simulink model "seldom_sim"  (R2024a)
settings: Solver=FixedStepAuto  StartTime=0.0  StopTime=30  FixedStep=framePeriod_s  RelTol=1e-9
values from neighbouring files (symbols this model uses):
  framePeriod_s = 1/frameRate_hz    (= 0.02)    [setup.m]
undefined symbols (not defined in the file or in its folder): accel_mps2, Aircraft, alt_wgs84_m, ch, current_ma, datetime, datevec, die_temp_c, Earth, Env, ext_gnss1, failsafe, fmu_imu, fmu_mag, frame_time_us, gps_tow_ms, gyro_radps, healthy, horz_acc_m, imu_healthy, inceptor, InitCond, installed, lat_rad, lon_rad, lost_frame, mag_ut, ned_vel_mps, new_data, num_sats, power_module, sys_time_us, Telem, vert_acc_m, voltage_v, week, WGS84
libraries: simulink x8, aerolibconvert2 x5, aerolibasang x3, aerolibtransform2 x2, aerolibgravity2 x2, aerolibatmos2 x1, sharedtransform x1, uavutilslib x1, vrlib x1, simulink_extras x1, spsLeadLagFilterLib x1, shared6dof x1
(part 2 of 2)

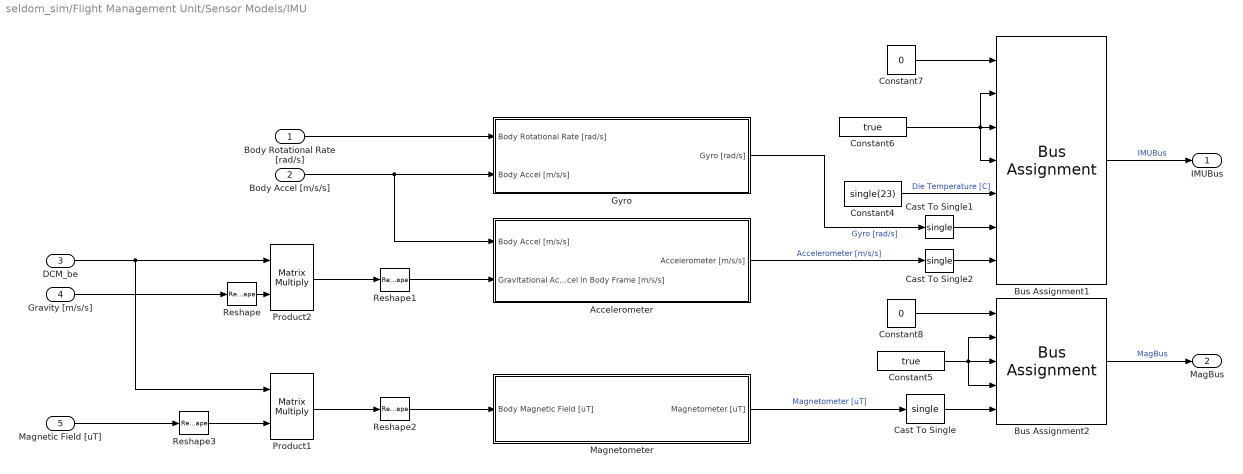
== system seldom_sim/Flight Management Unit/Sensor Models/IMU ==
  Body Rotational Rate [rad/s] : Inport
  Body Accel [m/s/s] : Inport  Port=2
  DCM_be : Inport  Port=3
  Gravity [m/s/s] : Inport  Port=4
  Magnetic Field [uT] : Inport  Port=5
  Accelerometer : Subsystem
  Bus Assignment1 : BusAssignment  AssignedSignals=installed,imu_healthy,new_data,die_temp_c,gyro_radps,accel_mps2
  Bus Assignment2 : BusAssignment  AssignedSignals=installed,healthy,new_data,mag_ut
  Cast To Single : DataTypeConversion  OutDataTypeStr=single  SaturateOnIntegerOverflow=off  RndMeth=Floor
  Cast To Single1 : DataTypeConversion  OutDataTypeStr=single  SaturateOnIntegerOverflow=off  RndMeth=Floor
  Cast To Single2 : DataTypeConversion  OutDataTypeStr=single  SaturateOnIntegerOverflow=off  RndMeth=Floor
  Constant4 : Constant  Value=single(23)
  Constant5 : Constant  Value=true
  Constant6 : Constant  Value=true
  Constant7 : Constant  Value=0  OutDataTypeStr=Bus: ImuData
  Constant8 : Constant  Value=0  OutDataTypeStr=Bus: MagData
  Gyro : Subsystem
  Magnetometer : Subsystem
  Product1 : Product  Multiplication=Matrix(*)
  Product2 : Product  Multiplication=Matrix(*)
  Reshape : Reshape  OutputDimensionality=Column vector (2-D)
  Reshape1 : Reshape
  Reshape2 : Reshape
  Reshape3 : Reshape  OutputDimensionality=Column vector (2-D)
  IMUBus : Outport
  MagBus : Outport  Port=2
  wires:
  Body Accel [m/s/s]/1 -> Accelerometer/1(Body Accel [m/s/s]), Gyro/2(Body Accel [m/s/s])
  DCM_be/1 -> Product1/1, Product2/1
  Gravity [m/s/s]/1 -> Reshape/1
  Product2/1 -> Reshape1/1
  Reshape1/1 -> Accelerometer/2(Gravitational Accel in Body Frame [m/s/s])
  Body Rotational Rate [rad/s]/1 -> Gyro/1(Body Rotational Rate [rad/s])
  Reshape2/1 -> Magnetometer/1(Body Magnetic Field [uT])
  Product1/1 -> Reshape2/1
  Reshape3/1 -> Product1/2
  Magnetic Field [uT]/1 -> Reshape3/1
  Magnetometer/1(Magnetometer [uT]) -> Cast To Single/1  "Magnetometer [uT]"
  Accelerometer/1(Accelerometer [m/s/s]) -> Cast To Single2/1  "Accelerometer [m/s/s]"
  Gyro/1(Gyro [rad/s]) -> Cast To Single1/1  "Gyro [rad/s]"
  Reshape/1 -> Product2/2
  Constant4/1 -> Bus Assignment1/5  "Die Temperature [C]"
  Constant7/1 -> Bus Assignment1/1
  Constant8/1 -> Bus Assignment2/1
  Bus Assignment2/1 -> MagBus/1  "MagBus"
  Bus Assignment1/1 -> IMUBus/1  "IMUBus"
  Constant5/1 -> Bus Assignment2/4, Bus Assignment2/2, Bus Assignment2/3
  Constant6/1 -> Bus Assignment1/4, Bus Assignment1/2, Bus Assignment1/3
  Cast To Single/1 -> Bus Assignment2/5
  Cast To Single1/1 -> Bus Assignment1/6
  Cast To Single2/1 -> Bus Assignment1/7

== system seldom_sim/Flight Management Unit/Sensor Models/MakeInceptorBus ==
  Inceptor : Inport
  Bus Assignment1 : BusAssignment  AssignedSignals=new_data,lost_frame,failsafe,ch
  Bus Selector2 : BusSelector  OutputSignals=New Data,Lost Frame,Failsafe,Channel Data
  Constant4 : Constant  Value=0  OutDataTypeStr=Bus: InceptorData
  InceptorBus : Outport
  wires:
  Bus Selector2/2 -> Bus Assignment1/3  "<Lost Frame>"
  Bus Selector2/1 -> Bus Assignment1/2  "<New Data>"
  Inceptor/1 -> Bus Selector2/1
  Bus Selector2/4 -> Bus Assignment1/5  "<Channel Data>"
  Bus Assignment1/1 -> InceptorBus/1  "InceptorBus"
  Bus Selector2/3 -> Bus Assignment1/4  "<Failsafe>"
  Constant4/1 -> Bus Assignment1/1

== system seldom_sim/Flight Management Unit/Sensor Models/MakePowerModuleBus ==
  Battery : Inport
  Bus Assignment1 : BusAssignment  AssignedSignals=voltage_v,current_ma
  Bus Selector2 : BusSelector  OutputSignals=Voltage [V],Current [V]
  Constant4 : Constant  Value=0  OutDataTypeStr=Bus: PowerModuleData
  PowerModuleBus : Outport
  wires:
  Constant4/1 -> Bus Assignment1/1
  Bus Assignment1/1 -> PowerModuleBus/1  "PowerModuleBus"
  Battery/1 -> Bus Selector2/1
  Bus Selector2/1 -> Bus Assignment1/2  "<Voltage [V]>"
  Bus Selector2/2 -> Bus Assignment1/3  "<Current [V]>"

== system seldom_sim/Flight Management Unit/Subsystem/Triggered Subsystem ==
  Wp : Inport
  Trigger : TriggerPort  VariantControl=(inherit)
  Constant : Constant  OutDataTypeStr=int16
  Sum : Sum  Inputs=|++  AccumDataTypeStr=uint16
  Wp++ : Outport
  wires:
  Wp/1 -> Sum/1
  Constant/1 -> Sum/2
  Sum/1 -> Wp++/1

== system seldom_sim/Vehicle/Forces and Moments/Aerodynamic ==
  note: In the future, the effect of blade flapping will be included. More experimental test need to be done to evaluate the v_forward to deflection angle constant in a wind tunnel.
  note: To calculate drag force, a look up table was created by recording the projected area at different incident angles. Assume the drone to resemble a cylinder (area changes as angle of attack changes, constant with sideslip changes)
  Dynamic Pressure : Inport
  body_vel : Inport  Port=2
  Calculate wind angle : Subsystem
  Cd : Constant  Value=Aircraft.Aero.Cd
  Drag contribution on moment : Constant  Value=[0 0 0]
  Drag in body frame : Product  Multiplication=Matrix(*)
  Gain : Gain  Gain=-1
  Mux1 : Mux  Inputs=2
  Normalize Vector : vrlib/Utilities/Normalize Vector  maxzero=0
  Product : Product  Inputs=3
  Radians to Degrees : simulink_extras/Transformations/Radians to Degrees
  Reshape : Reshape  OutputDimensionality=Row vector (2-D)
  alfa to frontal area look up table : Lookup_n-D  NumberOfTableDimensions=1  BreakpointsSpecification=Even spacing  BreakpointsForDimension1=[-90:10:90]  BreakpointsForDimension1FirstPoint=-180  BreakpointsForDimension1Spacing=10  Table=Aircraft.Geo.front_area_m2  InternalRulePriority=Speed  RndMeth=Simplest
  Fxyz Mxzy : Outport
  wires:
  Dynamic Pressure/1 -> Product/2
  Product/1 -> Drag in body frame/2
  Reshape/1 -> Fxyz Mxzy/1
  Mux1/1 -> Reshape/1
  Radians to Degrees/1 -> alfa to frontal area look up table/1
  alfa to frontal area look up table/1 -> Product/1  "Frontal area"
  Cd/1 -> Product/3
  Drag in body frame/1 -> Mux1/1
  Drag contribution on moment/1 -> Mux1/2
  Gain/1 -> Normalize Vector/1
  Normalize Vector/1 -> Drag in body frame/1
  body_vel/1 -> Gain/1, Calculate wind angle/1(body_vel_mps)
  Calculate wind angle/1(Incident_angle_rad) -> Radians to Degrees/1

== system seldom_sim/Vehicle/Forces and Moments/Gravitational ==
  Gravity [m/s/s] : Inport
  DCM_be : Inport  Port=2
  Gravity Moment : Constant  Value=[0 0 0]
  Mux : Mux  Inputs=2
  Product : Product
  Product1 : Product  Multiplication=Matrix(*)
  Reshape : Reshape  OutputDimensionality=Column vector (2-D)
  Reshape1 : Reshape
  UAV Mass : Constant  Value=Aircraft.Mass.mass_kg
  Fxyz Mxyz : Outport
  wires:
  UAV Mass/1 -> Product/2
  Product/1 -> Product1/2  "Gravity Force NED [N]"
  DCM_be/1 -> Product1/1
  Gravity Moment/1 -> Mux/2
  Mux/1 -> Fxyz Mxyz/1
  Reshape/1 -> Product/1
  Gravity [m/s/s]/1 -> Reshape/1
  Reshape1/1 -> Mux/1
  Product1/1 -> Reshape1/1  "Gravity Force Body [N]"

== system seldom_sim/Vehicle/Forces and Moments/Propulsive ==
  note: Should get replaced with full and proper motor lookup tables unless it is really very linear.
  note: Missing modeling of torque directly generated from the motor plus propeller spinning. Need to add that in.
  note: First order response model of motor thrust to command change.
  Motor Cmd : Inport
  Constant1 : Constant  Value=Aircraft.Motor.align
  Constant7 : Constant  Value=Aircraft.Motor.pos_m
  Demux1 : Demux  Outputs=3
  Demux2 : Demux  Outputs=3
  Gain : Gain  Gain=Aircraft.Motor.fmaxa_N
  Lead-Lag Filter : spsLeadLagFilterLib/Lead-Lag Filter  T1=0  T2=Aircraft.Motor.Tau  Vdc_Init=0  Ts=0
      settings: LibrarySourceBlock=|
      | sps_lib/Control/Filters/Lead-Lag
      | Filter
  Motor_Force_and_Moment_Body : MATLAB Function  TreatAsAtomicUnit=on
  Mux1 : Mux  Inputs=6
  PWM_norm : Subsystem
  Reshape2 : Reshape  OutputDimensionality=Row vector (2-D)
  Reshape3 : Reshape  OutputDimensionality=Row vector (2-D)
  Fxyz Mxyz : Outport
  wires:
  Reshape2/1 -> Motor_Force_and_Moment_Body/3(motor_thrust)
  Motor Cmd/1 -> PWM_norm/1(raw_sbus_in)
  Motor_Force_and_Moment_Body/2(Moment_motor) -> Demux1/1
  Demux1/1 -> Mux1/4  "Mx"
  Demux1/2 -> Mux1/5  "My"
  Constant7/1 -> Motor_Force_and_Moment_Body/1(motor_pos)
  Reshape3/1 -> Fxyz Mxyz/1
  Demux1/3 -> Mux1/6  "Mz"
  Mux1/1 -> Reshape3/1
  Constant1/1 -> Motor_Force_and_Moment_Body/2(motor_align)
  Demux2/2 -> Mux1/2  "Fy"
  Demux2/1 -> Mux1/1  "Fx"
  Demux2/3 -> Mux1/3  "Fz"
  Motor_Force_and_Moment_Body/1(Force_motor) -> Demux2/1
  Lead-Lag Filter/1 -> Gain/1  "PWM_ND_lag"
  Gain/1 -> Reshape2/1
  PWM_norm/1(normalized_out) -> Lead-Lag Filter/1  "PWM_ND"

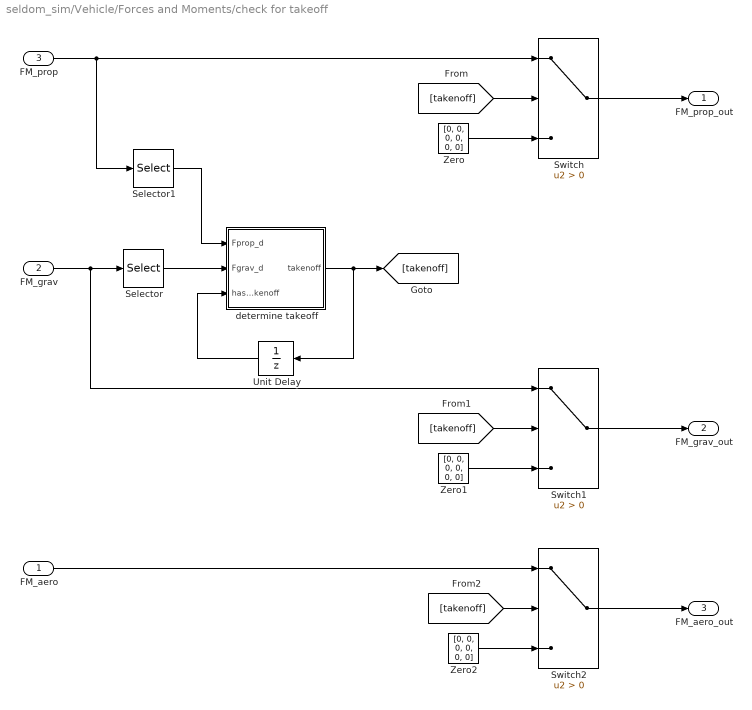
== system seldom_sim/Vehicle/Forces and Moments/check for takeoff ==
  FM_aero : Inport
  FM_grav : Inport  Port=2
  FM_prop : Inport  Port=3
  Selector : Selector  NumberOfDimensions=2  InputPortWidth=3  IndexOptions=Index vector (dialog),Index vector (dialog)  Indices=1,3  OutputSizes=1,1
  Selector1 : Selector  NumberOfDimensions=2  InputPortWidth=3  IndexOptions=Index vector (dialog),Index vector (dialog)  Indices=1,3  OutputSizes=1,1
  Switch : Switch  Criteria=u2 > Threshold  SaturateOnIntegerOverflow=off  InputSameDT=off
  Switch1 : Switch  Criteria=u2 > Threshold  SaturateOnIntegerOverflow=off  InputSameDT=off
  Switch2 : Switch  Criteria=u2 > Threshold  SaturateOnIntegerOverflow=off  InputSameDT=off
  Unit Delay : UnitDelay  InitialCondition=false  SampleTime=-1  HasFrameUpgradeWarning=on
  Zero : Constant  Value=[0, 0, 0, 0, 0, 0]  VectorParams1D=off  OutDataTypeStr=Inherit: Inherit via back propagation
  Zero1 : Constant  Value=[0, 0, 0, 0, 0, 0]  VectorParams1D=off  OutDataTypeStr=Inherit: Inherit via back propagation
  Zero2 : Constant  Value=[0, 0, 0, 0, 0, 0]  VectorParams1D=off  OutDataTypeStr=Inherit: Inherit via back propagation
  determine takeoff : Subsystem
  FM_prop_out : Outport
  FM_grav_out : Outport  Port=2
  FM_aero_out : Outport  Port=3
  wires:
  Switch2/1 -> FM_aero_out/1
  [takenoff] -> Switch1/2
  FM_prop/1 -> Selector1/1, Switch/1
  FM_aero/1 -> Switch2/1
  Switch1/1 -> FM_grav_out/1
  Selector1/1 -> determine takeoff/1(Fprop_d)
  FM_grav/1 -> Selector/1, Switch1/1
  Unit Delay/1 -> determine takeoff/3(has_takenoff)
  determine takeoff/1(takenoff) -> [takenoff], Unit Delay/1
  Zero1/1 -> Switch1/3
  Zero2/1 -> Switch2/3
  Zero/1 -> Switch/3
  Selector/1 -> determine takeoff/2(Fgrav_d)
  [takenoff] -> Switch/2
  [takenoff] -> Switch2/2
  Switch/1 -> FM_prop_out/1

== system seldom_sim/Vehicle/Vehicle Model/Norm ==
  2D Vector : Inport
  Product : Product
  Sqrt : Sqrt
  Sum of Elements : Sum  Inputs=+
  Norm : Outport
  wires:
  2D Vector/1 -> Product/2, Product/1
  Product/1 -> Sum of Elements/1
  Sum of Elements/1 -> Sqrt/1
  Sqrt/1 -> Norm/1

== system seldom_sim/Vehicle/Vehicle Model/determine airespeed ==
  Vb : Inport
  Compare To Constant : simulink/Logic and Bit Operations/Compare To Constant  relop=>  const=0  OutDataTypeStr=boolean
  MatrixMultiply : Product  Multiplication=Matrix(*)
  Reshape : Reshape  OutputDimensionality=Column vector (2-D)
  Reshape1 : Reshape  OutputDimensionality=Row vector (2-D)
  Subsystem : Subsystem
  AoA rate : Outport
  Alpha : Outport  Port=2
  Beta : Outport  Port=3
  beta rate : Outport  Port=4
  airspeed : Outport  Port=5
  wires:
  Vb/1 -> Subsystem/1(Vb), Reshape/1, Reshape1/1
  Reshape1/1 -> MatrixMultiply/1
  Reshape/1 -> MatrixMultiply/2
  MatrixMultiply/1 -> Compare To Constant/1
  Subsystem/1(AoA rate) -> AoA rate/1
  Subsystem/2(Alpha) -> Alpha/1
  Subsystem/3(Beta) -> Beta/1
  Subsystem/4(beta rate) -> beta rate/1
  Subsystem/5(V) -> airspeed/1
  Compare To Constant/1 -> Subsystem/Enable

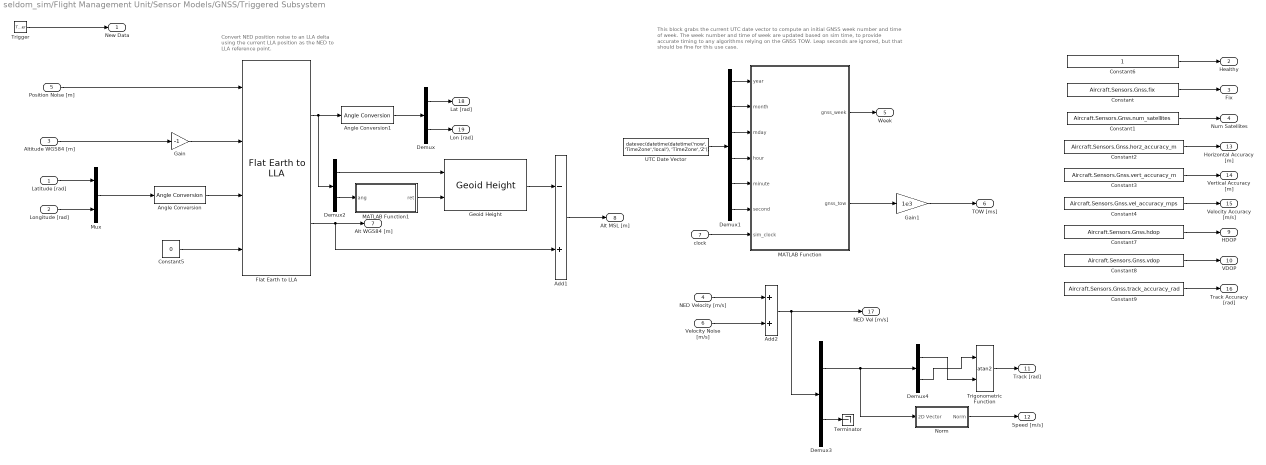
== system seldom_sim/Flight Management Unit/Sensor Models/GNSS/Triggered Subsystem ==
  note: This block grabs the current UTC date vector to compute an initial GNSS week number
      | and time of week. The week number and time of week are updated based on sim time, to provide accurate timing to any algorithms relying on the GNSS TOW. Leap seconds are ignored, but that should be fine for this use case.
  note: Convert NED position noise to an LLA delta
      | using the current LLA position as the NED to
      | LLA reference point.
  Latitude [rad] : Inport
  "Longitude [rad] " : Inport  Port=2
  Altitude WGS84 [m] : Inport  Port=3
  NED Velocity [m/s] : Inport  Port=4  PortDimensions=3
  Position Noise [m] : Inport  Port=5  PortDimensions=3
  Velocity Noise [m/s] : Inport  Port=6  PortDimensions=3
  clock : Inport  Port=7
  Trigger : TriggerPort  VariantControl=Variant  ShowOutputPort=on  OutputDataType=int8
  Add1 : Sum  Inputs=-+
  Add2 : Sum
  Angle Conversion : aerolibconvert2/Angle Conversion  IU=rad  OU=deg
  Angle Conversion1 : aerolibconvert2/Angle Conversion  IU=deg  OU=rad
  Constant : Constant  Value=Aircraft.Sensors.Gnss.fix
  Constant1 : Constant  Value=Aircraft.Sensors.Gnss.num_satellites
  Constant2 : Constant  Value=Aircraft.Sensors.Gnss.horz_accuracy_m
  Constant3 : Constant  Value=Aircraft.Sensors.Gnss.vert_accuracy_m
  Constant4 : Constant  Value=Aircraft.Sensors.Gnss.vel_accuracy_mps
  Constant5 : Constant  Value=0
  Constant6 : Constant
  Constant7 : Constant  Value=Aircraft.Sensors.Gnss.hdop
  Constant8 : Constant  Value=Aircraft.Sensors.Gnss.vdop
  Constant9 : Constant  Value=Aircraft.Sensors.Gnss.track_accuracy_rad
  Demux : Demux  Outputs=2
  Demux1 : Demux  Outputs=6
  Demux2 : Demux  Outputs=2
  Demux3 : Demux  Outputs=[2 1]
  Demux4 : Demux  Outputs=2
  Flat Earth to LLA : aerolibtransform2/Flat Earth to LLA  units=Metric (MKS)  ptype=Earth (WGS84)  F=1/298.257223563  R=6378137  refPosPort=on  LL0=[0 10]  psi=0
  Gain : Gain  Gain=-1
  Gain1 : Gain  Gain=1e3
  Geoid Height : aerolibgravity2/Geoid Height  units=Metric (MKS)  gtype=EGM96  datafile='geoidegm96grid'  dtype=double  action=Warning
  MATLAB Function : MATLAB Function  TreatAsAtomicUnit=on
  MATLAB Function1 : MATLAB Function  TreatAsAtomicUnit=on
  Mux : Mux  Inputs=2
  Norm : Subsystem
  Terminator : Terminator
  Trigonometric Function : Trigonometry  Operator=atan2
  UTC Date Vector : Constant  Value=datevec(datetime(datetime('now', 'TimeZone','local'), 'TimeZone','Z'))  SampleTime=-1
  New Data : Outport
  Healthy : Outport  Port=2
  Fix : Outport  Port=3
  Num Satellites : Outport  Port=4
  Week : Outport  Port=5
  TOW [ms] : Outport  Port=6
  Alt WGS84 [m] : Outport  Port=7
  Alt MSL [m] : Outport  Port=8
  HDOP : Outport  Port=9
  VDOP : Outport  Port=10
  Track [rad] : Outport  Port=11
  Speed [m/s] : Outport  Port=12
  Horizontal Accuracy [m] : Outport  Port=13
  Vertical Accuracy [m] : Outport  Port=14
  Velocity Accuracy [m/s] : Outport  Port=15
  Track Accuracy [rad] : Outport  Port=16
  NED Vel [m/s] : Outport  Port=17
  Lat [rad] : Outport  Port=18
  Lon [rad] : Outport  Port=19
  wires:
  Constant/1 -> Fix/1
  Constant1/1 -> Num Satellites/1
  Constant2/1 -> Horizontal Accuracy [m]/1
  Constant3/1 -> Vertical Accuracy [m]/1
  Constant4/1 -> Velocity Accuracy [m/s]/1
  Position Noise [m]/1 -> Flat Earth to LLA/1
  Altitude WGS84 [m]/1 -> Gain/1
  Mux/1 -> Angle Conversion/1
  Angle Conversion/1 -> Flat Earth to LLA/3
  Constant5/1 -> Flat Earth to LLA/4
  "Longitude [rad] "/1 -> Mux/2
  Latitude [rad]/1 -> Mux/1
  Flat Earth to LLA/1 -> Demux2/1, Angle Conversion1/1
  Angle Conversion1/1 -> Demux/1
  Demux/2 -> Lon [rad]/1
  Demux/1 -> Lat [rad]/1
  Flat Earth to LLA/2 -> Add1/2, Alt WGS84 [m]/1
  NED Velocity [m/s]/1 -> Add2/1
  Add2/1 -> Demux3/1, NED Vel [m/s]/1
  Demux1/2 -> MATLAB Function/2(month)
  Demux1/6 -> MATLAB Function/6(second)
  UTC Date Vector/1 -> Demux1/1
  Demux1/1 -> MATLAB Function/1(year)
  Demux1/5 -> MATLAB Function/5(minute)
  Demux1/4 -> MATLAB Function/4(hour)
  Demux1/3 -> MATLAB Function/3(mday)
  MATLAB Function/2(gnss_tow) -> Gain1/1
  MATLAB Function/1(gnss_week) -> Week/1
  clock/1 -> MATLAB Function/7(sim_clock)
  Gain/1 -> Flat Earth to LLA/2
  Constant6/1 -> Healthy/1
  Trigger/1 -> New Data/1
  Gain1/1 -> TOW [ms]/1
  Demux2/1 -> Geoid Height/1
  Demux2/2 -> MATLAB Function1/1(ang)
  MATLAB Function1/1(ret) -> Geoid Height/2
  Geoid Height/1 -> Add1/1
  Add1/1 -> Alt MSL [m]/1
  Constant7/1 -> HDOP/1
  Constant8/1 -> VDOP/1
  Demux4/1 -> Trigonometric Function/2
  Demux4/2 -> Trigonometric Function/1
  Trigonometric Function/1 -> Track [rad]/1
  Velocity Noise [m/s]/1 -> Add2/2
  Constant9/1 -> Track Accuracy [rad]/1
  Demux3/1 -> Norm/1(2D Vector), Demux4/1
  Demux3/2 -> Terminator/1
  Norm/1(Norm) -> Speed [m/s]/1

== system seldom_sim/Flight Management Unit/Sensor Models/IMU/Accelerometer ==
  Body Accel [m/s/s] : Inport  PortDimensions=3
  Gravitational Accel in Body Frame [m/s/s] : Inport  Port=2  PortDimensions=3
  Add : Sum  Inputs=+++
  Band-Limited White Noise : simulink/Sources/Band-Limited White Noise  Cov=Aircraft.Sensors.Imu.Accel.noise_mps2  Ts=0.1  seed=[23341]
  Constant : Constant  Value=Aircraft.Sensors.Imu.Accel.bias_mps2  VectorParams1D=off
  Constant1 : Constant  Value=Aircraft.Sensors.Imu.Accel.scale_factor
  Product : Product  Multiplication=Matrix(*)
  Reshape : Reshape  OutputDimensionality=Column vector (2-D)
  Reshape1 : Reshape  OutputDimensionality=Column vector (2-D)
  Reshape2 : Reshape
  Saturation : Saturate  UpperLimit=Aircraft.Sensors.Imu.Accel.upper_limit_mps2  LowerLimit=Aircraft.Sensors.Imu.Accel.lower_limit_mps2
  Subtract : Sum  Inputs=+-
  Accelerometer [m/s/s] : Outport  PortDimensions=3
  wires:
  Add/1 -> Saturation/1
  Band-Limited White Noise/1 -> Add/1
  Product/1 -> Add/3
  Constant/1 -> Add/2
  Constant1/1 -> Product/1
  Subtract/1 -> Product/2
  Reshape/1 -> Subtract/2
  Gravitational Accel in Body Frame [m/s/s]/1 -> Reshape/1
  Reshape1/1 -> Subtract/1
  Body Accel [m/s/s]/1 -> Reshape1/1
  Saturation/1 -> Reshape2/1
  Reshape2/1 -> Accelerometer [m/s/s]/1

== system seldom_sim/Flight Management Unit/Sensor Models/IMU/Gyro ==
  Body Rotational Rate [rad/s] : Inport  PortDimensions=3
  Body Accel [m/s/s] : Inport  Port=2  PortDimensions=3
  Add1 : Sum  Inputs=++++
  Band-Limited White Noise : simulink/Sources/Band-Limited White Noise  Cov=Aircraft.Sensors.Imu.Gyro.noise_radps  Ts=0.1  seed=[23341]  VectorParams1D=off
  Constant1 : Constant  Value=Aircraft.Sensors.Imu.Gyro.bias_radps  VectorParams1D=off
  Constant2 : Constant  Value=Aircraft.Sensors.Imu.Gyro.accel_sens_radps
  Constant3 : Constant  Value=Aircraft.Sensors.Imu.Gyro.scale_factor  VectorParams1D=off
  Product : Product
  Product1 : Product  Multiplication=Matrix(*)
  Reshape : Reshape  OutputDimensionality=Column vector (2-D)
  Reshape1 : Reshape  OutputDimensionality=Column vector (2-D)
  Reshape2 : Reshape
  Saturation : Saturate  UpperLimit=Aircraft.Sensors.Imu.Gyro.upper_limit_radps  LowerLimit=Aircraft.Sensors.Imu.Gyro.lower_limit_radps
  Gyro [rad/s] : Outport  PortDimensions=3
  wires:
  Constant3/1 -> Product1/1
  Constant2/1 -> Product/1
  Add1/1 -> Saturation/1
  Constant1/1 -> Add1/3
  Product1/1 -> Add1/4
  Band-Limited White Noise/1 -> Add1/2
  Body Rotational Rate [rad/s]/1 -> Reshape/1
  Reshape/1 -> Product1/2
  Body Accel [m/s/s]/1 -> Product/2
  Product/1 -> Reshape1/1
  Reshape1/1 -> Add1/1
  Reshape2/1 -> Gyro [rad/s]/1
  Saturation/1 -> Reshape2/1

== system seldom_sim/Flight Management Unit/Sensor Models/IMU/Magnetometer ==
  Body Magnetic Field [uT] : Inport  PortDimensions=3
  Add2 : Sum  Inputs=+++
  Band-Limited White Noise : simulink/Sources/Band-Limited White Noise  Cov=Aircraft.Sensors.Imu.Mag.noise_ut  Ts=0.1  seed=[23341]
  Constant1 : Constant  Value=Aircraft.Sensors.Imu.Mag.scale_factor  VectorParams1D=off
  Constant2 : Constant  Value=Aircraft.Sensors.Imu.Mag.bias_ut
  Product : Product  Multiplication=Matrix(*)
  Reshape : Reshape  OutputDimensionality=Column vector (2-D)
  Reshape1 : Reshape
  Saturation : Saturate  UpperLimit=Aircraft.Sensors.Imu.Mag.upper_limit_ut  LowerLimit=Aircraft.Sensors.Imu.Mag.lower_limit_ut
  Magnetometer [uT] : Outport  PortDimensions=3
  wires:
  Body Magnetic Field [uT]/1 -> Reshape/1
  Band-Limited White Noise/1 -> Add2/1
  Add2/1 -> Saturation/1
  Constant2/1 -> Add2/2
  Constant1/1 -> Product/1
  Reshape/1 -> Product/2
  Saturation/1 -> Reshape1/1
  Reshape1/1 -> Magnetometer [uT]/1
  Product/1 -> Add2/3

== system seldom_sim/Vehicle/Forces and Moments/Aerodynamic/Calculate wind angle ==
  body_vel_mps : Inport
  calculate_wind_angle : MATLAB Function  TreatAsAtomicUnit=on
  Incident_angle_rad : Outport
  wires:
  body_vel_mps/1 -> calculate_wind_angle/1(body_vel)
  calculate_wind_angle/1(inc_ang) -> Incident_angle_rad/1

== system seldom_sim/Vehicle/Forces and Moments/Propulsive/PWM_norm ==
  raw_sbus_in : Inport
  Constant : Constant  Value=Aircraft.PWM.norm_min  OutDataTypeStr=single
  Constant1 : Constant  Value=Aircraft.PWM.min  OutDataTypeStr=single
  Constant2 : Constant  Value=Aircraft.PWM.max  OutDataTypeStr=single
  Constant3 : Constant  Value=Aircraft.PWM.norm_max  OutDataTypeStr=single
  remap : MATLAB Function  TreatAsAtomicUnit=on
  normalized_out : Outport
  wires:
  Constant3/1 -> remap/5(out_max)
  Constant/1 -> remap/4(out_min)
  Constant2/1 -> remap/3(in_max)
  Constant1/1 -> remap/2(in_min)
  remap/1(norm_out) -> normalized_out/1
  raw_sbus_in/1 -> remap/1(raw_in)

== system seldom_sim/Vehicle/Forces and Moments/check for takeoff/determine takeoff ==
  Fprop_d : Inport
  Fgrav_d : Inport  Port=2
  has_takenoff : Inport  Port=3
  Gain : Gain  Gain=-1
  GreaterThan : RelationalOperator  Operator=>  OutDataTypeStr=boolean  RndMeth=Simplest  InputSameDT=off
  OR : Logic  Operator=OR  IconShape=distinctive  AllPortsSameDT=off  OutDataTypeStr=boolean
  takenoff : Outport
  wires:
  Fgrav_d/1 -> GreaterThan/2
  Fprop_d/1 -> Gain/1
  Gain/1 -> GreaterThan/1
  GreaterThan/1 -> OR/1
  has_takenoff/1 -> OR/2
  OR/1 -> takenoff/1

== system seldom_sim/Vehicle/Vehicle Model/determine airespeed/Subsystem ==
  Vb : Inport
  Enable : EnablePort  StatesWhenEnabling=reset
  Derivative : Derivative
  Derivative1 : Derivative
  "Incidence, Sideslip, & Airspeed" : aerolibasang/Incidence, Sideslip, & Airspeed
  AoA rate : Outport
  Alpha : Outport  Port=2
  Beta : Outport  Port=3
  beta rate : Outport  Port=4
  V : Outport  Port=5
  wires:
  Derivative1/1 -> beta rate/1
  Vb/1 -> "Incidence, Sideslip, & Airspeed"/1
  "Incidence, Sideslip, & Airspeed"/2 -> Beta/1, Derivative1/1
  "Incidence, Sideslip, & Airspeed"/3 -> V/1
  "Incidence, Sideslip, & Airspeed"/1 -> Alpha/1, Derivative/1
  Derivative/1 -> AoA rate/1

== system seldom_sim/Flight Management Unit/Sensor Models/GNSS/Triggered Subsystem/Norm ==
  2D Vector : Inport
  Product : Product
  Sqrt : Sqrt
  Sum of Elements : Sum  Inputs=+
  Norm : Outport
  wires:
  2D Vector/1 -> Product/2, Product/1
  Product/1 -> Sum of Elements/1
  Sum of Elements/1 -> Sqrt/1
  Sqrt/1 -> Norm/1

== matlab function seldom_sim/Pilot Input/estop/remap ==
  data: raw_in input; norm_out output; in_min input; in_max input; out_min input; out_max input
function norm_out = remap(raw_in,in_min,in_max,out_min,out_max)
norm_out = (raw_in - in_min) * (out_max - out_min)/(in_max-in_min) + out_min;

== matlab function seldom_sim/Pilot Input/mode/remap ==
  data: raw_in input; norm_out output; in_min input; in_max input; out_min input; out_max input
function norm_out = remap(raw_in,in_min,in_max,out_min,out_max)
norm_out = (raw_in - in_min) * (out_max - out_min)/(in_max-in_min) + out_min;

== matlab function seldom_sim/Pilot Input/roll_rate_cmd/remap ==
  data: raw_in input; norm_out output; in_min input; in_max input; out_min input; out_max input
function norm_out = remap(raw_in,in_min,in_max,out_min,out_max)
norm_out = (raw_in - in_min) * (out_max - out_min)/(in_max-in_min) + out_min;

== matlab function seldom_sim/Pilot Input/pitch_rate_cmd/remap ==
  data: raw_in input; norm_out output; in_min input; in_max input; out_min input; out_max input
function norm_out = remap(raw_in,in_min,in_max,out_min,out_max)
norm_out = (raw_in - in_min) * (out_max - out_min)/(in_max-in_min) + out_min;

== matlab function seldom_sim/Vehicle/Vehicle Model/MATLAB Function ==
  data: ang input; ret output
function ret  = constrain360(ang)
%Constrain360 Converts a +/-180 value to a 0 - 360 value
ret = fmod(ang, 360);
if ret < 0
    ret = ret + 360;
end

end

== matlab function seldom_sim/Pilot Input/yaw_rate_cmd/remap ==
  data: raw_in input; norm_out output; in_min input; in_max input; out_min input; out_max input
function norm_out = remap(raw_in,in_min,in_max,out_min,out_max)
norm_out = (raw_in - in_min) * (out_max - out_min)/(in_max-in_min) + out_min;

== matlab function seldom_sim/Flight Management Unit/Sensor Models/GNSS/Triggered Subsystem/MATLAB Function ==
  data: year input; month input; mday input; hour input; minute input; second input; gnss_week output; sim_clock input; gnss_tow output
function [gnss_week, gnss_tow] = GnssWeekAndTime(year, month, mday, hour, minute, second, sim_clock)

JAN61980 = 44244;
JAN11901 = 15385;
SEC_PER_DAY = 86400.0;

month_day = [
    0, 31, 59, 90, 120, 151, 181, 212, 243, 273, 304, 334;
    0, 31, 60, 91, 121, 152, 182, 213, 244, 274, 305, 335
];

second = second + sim_clock;
leap = (mod(year,4) == 0);
yday = month_day(leap + 1, month) + mday;
mjd = ((year - 1901) / 4) * 1461 + mod((year - 1901), 4) * 365 + yday - 1 + JAN11901;
fmjd = ((second / 60.0 + minute) / 60.0 + hour) / 24.0;
gnss_week = floor((mjd - JAN61980) / 7);
gnss_tow = ((mjd - JAN61980) - gnss_week * 7 + fmjd) * SEC_PER_DAY;

== matlab function seldom_sim/Flight Management Unit/Sensor Models/GNSS/Triggered Subsystem/MATLAB Function1 ==
  data: ang input; ret output
function ret  = constrain360(ang)
%Constrain360 Converts a +/-180 value to a 0 - 360 value
ret = fmod(ang, 360);
if ret < 0
    ret = ret + 360;
end

end

== matlab function seldom_sim/Vehicle/Forces and Moments/Aerodynamic/Calculate wind angle/calculate_wind_angle ==
  data: body_vel input; inc_ang output
function inc_ang = calculate_wind_angle(body_vel)

xy_mag = norm(body_vel(1:2));
if xy_mag > 0
    inc_ang = atan(xy_mag / body_vel(3));
else
    inc_ang = 0;
end

== matlab function seldom_sim/Pilot Input/VelU_cmd/remap ==
  data: raw_in input; norm_out output; in_min input; in_max input; out_min input; out_max input
function norm_out = remap(raw_in,in_min,in_max,out_min,out_max)
norm_out = (raw_in - in_min) * (out_max - out_min)/(in_max-in_min) + out_min;

== matlab function seldom_sim/Pilot Input/VelN_cmd/remap ==
  data: raw_in input; norm_out output; in_min input; in_max input; out_min input; out_max input
function norm_out = remap(raw_in,in_min,in_max,out_min,out_max)
norm_out = (raw_in - in_min) * (out_max - out_min)/(in_max-in_min) + out_min;

== matlab function seldom_sim/Vehicle/Forces and Moments/Propulsive/Motor_Force_and_Moment_Body ==
  data: Force_motor output; motor_pos input; motor_align input; motor_thrust input; Moment_motor output
function [Force_motor,Moment_motor] = thrust_to_moment(motor_pos,motor_align,motor_thrust)
% Properly apply each motor's thrust to the correct orientation, then
% calculate the moment generated by each motor thrust
nmotor = numel(motor_thrust);
Force_motor_temp = zeros (nmotor,3);
Moment_motor_temp = zeros (nmotor,3);
for i = 1:nmotor
    Force_motor_temp(i,:) = motor_thrust(i)*motor_align(i,:); % F = T*normal_unit_vec
    Moment_motor_temp(i,:) = motor_thrust(i)*cross(motor_pos(i,:),motor_align(i,:)); % M = T*(pos-CG cross normal_unit_vec)
end
Force_motor  = sum (Force_motor_temp);
Moment_motor = sum (Moment_motor_temp);
end

== matlab function seldom_sim/Vehicle/Forces and Moments/Propulsive/PWM_norm/remap ==
  data: raw_in input; norm_out output; in_min input; in_max input; out_min input; out_max input
function norm_out = remap(raw_in,in_min,in_max,out_min,out_max)
norm_out = (raw_in - in_min) * (out_max - out_min)/(in_max-in_min) + out_min;

== matlab function seldom_sim/Pilot Input/VelE_cmd/remap ==
  data: raw_in input; norm_out output; in_min input; in_max input; out_min input; out_max input
function norm_out = remap(raw_in,in_min,in_max,out_min,out_max)
norm_out = (raw_in - in_min) * (out_max - out_min)/(in_max-in_min) + out_min;
